simulink model "VMO_GP"  (R2021a)
settings: Solver=VariableStepAuto  StartTime=0.0  StopTime=50  FixedStep=0.001  RelTol=1e-3
model workspace (MAT data in the model file):
  lambda = 20
  po = [0  0  0.5; 0.5  0  0; 0  0  -0.5; -0.5  0  0]
undefined symbols (not defined in the file or in its folder): mergepose
libraries: simlib_vpc_basic x4, simlib_vpc_coremath x2, simlib_vpc_gp x1
settings Model: Creator=marco  LastModifiedBy=marco
settings SolverCC: AlgebraicLoopSolver=TrustRegion
settings DebuggingCC: AlgebraicLoopMsg=none  SFMachineParentedDataDiag=warning
settings RTWCC: Toolchain=Clang v3.1 | gmake (64-bit Mac)

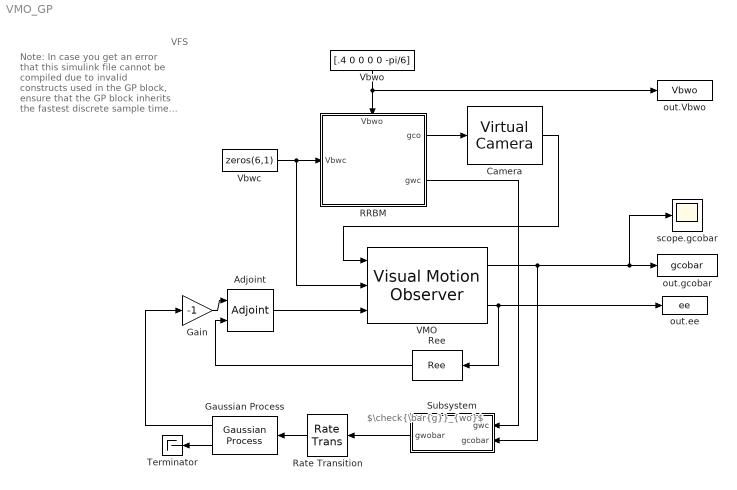
== system VMO_GP ==
  note: VFS
  note: $\check{\bar{g}}_{wo}$
  note: Note:
      |
      | In case you get an error that this simulink file cannot be compiled due to invalid constructs used in the GP block, ensure that the GP block inherits the fastest discrete sample time if you use a variable step solver!
      |
      | Simulink sometimes tends to forget this setting if the file has been altered by library block updates...
  Adjoint : simlib_vpc_basic/Adjoint  adjointtype=orientation
      settings: SourceProductName=VPC Library
  Camera : simlib_vpc_basic/Virtual Camera  camtype=Pinhole  po=po  lambda=lambda
      settings: SourceProductName=VPC Library
  Gain : Gain  Gain=-1
  Gaussian Process : simlib_vpc_gp/Gaussian Process  X=[0.630556779825130,-1.35266887136097,0.100000000000000,0,0,-2.69410960293706;-0.463678144695271,-0.643799212064173,0.100000000000000,0,0,1.54442416387410;0.824727377358984,-1.21916548494542,0.100000000000000,0,0,-2.38442385676060;-0.452218900404542,-0.797273527670285,0.100000000000000,0,0,1.74622300936847;0.0735614873622379,-1.39355710178978,0.100000000000000,0,0,2.84066394855618;1.02709161361236,-0.429534249029276,0.100000000000000,0,0,-1.25892388595008;0.466856822301989,0.0815553296307524,0.100000000000000,0,0,-0.220190026018465;0.700684091841969,-0.0135113083777034,0.100000000000000,0,0,-0.552120963315916;-0.371594765405859,-0.299841291908943,0.100000000000000,0,0,1.07400302698064;0.493112507590971,0.0751893431225574,0.100000000000000,0,0,-0.255556274277872;0.281774950670647,-1.42767003232909,0.100000000000000,0,0,3.11773385638550;0.454855984665292,0.0841403324164895,0.100000000000000,0,0,-0.204120492121210;-0.415643299934273,-0.931272694722223,0.100000000000000,0,0,1.92829566524218;-0.463704413816322,-0.644822651287869,0.100000000000000,0,0,1.54576428394557;0.556071793384051,0.0558043832070477,0.100000000000000,0,0,-0.341814497897213;0.693810642313243,-1.31856056106307,0.100000000000000,0,0,-2.60000519109390;0.139429262029952,-1.41082195312738,0.100000000000000,0,0,2.92982683484421;0.225444734023850,-1.42424078855668,0.100000000000000,0,0,3.04384446142033;0.336503259664140,0.0991274476359257,0.100000000000000,0,0,-0.0478008530352022;-0.0531708161840424,-1.34135090449317,0.100000000000000,0,0,2.66100597056373]  Y=[0.400400483777776,6.20811263679909e-05,-0.000162652488464400,-0.000273446486135386,-0.000116687704346113,-0.523637613189225;0.399798663298112,6.11577178236449e-05,-1.83837233443192e-05,-5.72316425158164e-06,6.14391667114607e-05,-0.523595018762085;0.399925527207886,0.000102384004761238,-1.86739670271565e-05,-7.65017896653280e-06,1.02416118127720e-05,-0.523520368962881;0.399947525768678,-1.43211998020437e-05,3.27587119859464e-05,0.000113295220747682,-3.51700486357816e-05,-0.523531017064327;0.400111825354472,3.90999913623867e-05,5.26454668989892e-05,-9.40761215372331e-06,-4.25671711451752e-05,-0.523522634661440;0.399825833671039,-7.77258024196419e-05,-0.000206163047832629,6.59457899046355e-06,-8.22951844090592e-05,-0.523698419763352;0.399974962089588,-1.88854060648864e-05,3.09965613525548e-05,0.000245980243067202,-0.000217647213137394,-0.523689484439025;0.400074095697642,-1.41829641564855e-05,4.84335658930588e-05,4.75025873122616e-05,-9.10729403185158e-05,-0.523588569617585;0.400083248675279,0.000132443300246046,-0.000157442907631115,-2.83480572397296e-05,-4.51136693628445e-07,-0.523633397263088;0.400032876833907,6.44379360130703e-05,-0.000128770670171243,1.64273840062151e-05,-5.42887023463567e-05,-0.523597545840270;0.399861552080262,4.56874083328404e-06,7.00785975750203e-05,-6.15101314259443e-07,4.31078905663889e-05,-0.523618963169823;0.399914551858832,-2.55383556669599e-05,-1.30390132312550e-06,7.61551335297795e-05,6.91286456425908e-05,-0.523720317431230;0.399989694796018,-9.69835284456510e-05,-0.000159624446683547,5.99762161919923e-05,0.000131711278614893,-0.523655772898916;0.400222298778977,-0.000246033432409541,0.000124299539566767,-0.000133706441116990,-2.05671749582727e-05,-0.523700638665687;0.399762190818026,-6.58016860859998e-05,-0.000101273579864964,-4.49734662190949e-05,-4.24077389374409e-05,-0.523699857561119;0.399890067610248,8.46601373619946e-05,0.000103500553198445,2.49750235544482e-05,-0.000122935827076731,-0.523757337794273;0.400083233949163,-8.14595746369251e-05,6.44687411206958e-05,-3.23632580436771e-05,5.02141191648383e-05,-0.523497516354906;0.400296665626679,4.06352239193496e-05,1.07765346007298e-05,9.65656080285521e-05,-6.27072577361815e-05,-0.523553573528897;0.400010008726827,-1.62468044620332e-06,-9.59528973827606e-06,-0.000138103359704066,1.33199410225313e-05,-0.523641337975467;0.400029450602431,-0.000122327126645188,0.000161646482165890,-0.000230740252290899,7.19352758249854e-05,-0.523425710873170]  sigman=1e-2.*ones(6,1)  kernel=Squared Exponential ARD  hyp=[168349.386723878,4375.40145868387,1,1,1,479344.764312913,0.399829624229871;28.6402467014848,24.0814787639094,1,1,1,805.684470437413,2.45252270103894e-11;108.279817332599,159.557667315089,1,1,1,114449.667169593,3.58973817196935e-12;36.4794037030670,12.8797220031653,1,1,1,5438.09149501526,4.41867700247680e-09;2.19447546863541,62.6618892840448,1,1,1,8349.10365718305,1.24554979865875e-05;6611001.04652391,10465.6546012474,1,1,1,35776.6715743359,0.523405437753361]
      settings: SourceProductName=VPC Library
  RRBM : Subsystem
      settings: PortSchema="{\"entries\":[{\"content\":{\"sides\":[{\"content\":{\"connectorIds\":[\"In1\"]},\"type\":\"ConnectorPlacement.EquallySpacedRectSide\",\"uuid\":\"ce1006a6-ff18-4db7-ad69-3a60144a672f\"},{\"content\":{\"connectorIds\":[\"Out1\",\"Out2\"],\"side\":\"RIGHT\"},\"type\":\"ConnectorPlacement.EquallySpacedRectSide\",\"uuid\":\"9f6b7cf2-eb23-4db0-862a-f9244538bf77\"},{\"content\":{\"connectorIds\":[\"In2\"],\"side\":\"TOP\"},\"type\":\"ConnectorPlacement.EquallySpacedRectSide\",\"uuid\":\"e4abfdaf-0145-4439-9abb-46234dad4713\"},{\"content\":{\"connectorIds\":[],\"side\":\"HIDDEN\"},\"type\":\"ConnectorPlacement.EquallySpacedRectSide\",\"uuid\":\"77f0040d-d5e2-4b47-95e1-996605172696\"}]},\"type\":\"ConnectorPlacement.EquallySpacedConnector\",\"uuid\":\"a30e6cf8-5cfd-45cc-9c7f-0b16cc268ba1\"}],\"packageUris\":[\"http://schema.mathworks.com/mf0/Connector/R2020b\"],\"version\":\"1.0\"}"
      mask Display:
      | % Glitch in Matlab: If you define a line whose starting point and end point
      | % is equal, then the entire mask block is plotted in bold
      | plot([0,0],[0,0])
      | 
      | % Draw Box
      | plot([0,1,1,0,0],[0,0,1,1,0])
      | 
      | % Write label
      | fprintf('1 Agent\n1 Target','texmode','on')
      | 
      | % Label ports
      | port_label('input',1,'V^{b}_{wc}','texmode','on')
      | port_label('input',2,'V^{b}_{wo}','texmode','on')
      | port_label('output',1,'g_{co}','texmode','on')
      | port_label('output',2,'g_{wc}','texmode','on')
  Rate Transition : RateTransition
  Ree : simlib_vpc_coremath/Ree
      settings: SourceProductName=VPC Library
  Subsystem : Subsystem
      mask Display:
      | % Write label
      | % disp('Trans','texmode','on')
      | 
      | % Label ports
      | port_label('input',1,'g_{wc}','texmode','on')
      | port_label('input',2,'g_{co,bar}','texmode','on')
      | port_label('output',1,'g^{\upsilon}_{wo,bar}','texmode','on')
  Terminator : Terminator
  VMO : simlib_vpc_basic/Visual Motion Observer  gcobar0=mergepose(eye(3),[0 1 0])  projection=on  Ke_source=internal  Ke=5*eye(6)  show_ue_aux=on  show_ee=on  show_dgcobar=off  camtype=Pinhole  fo=po  lambda=lambda
      settings: SourceProductName=VPC Library
  Vbwc : Constant  Value=zeros(6,1)
  Vbwo : Constant  Value=[.4 0 0 0 0 -pi/6]
  out.Vbwo : ToWorkspace  VariableName=Vbwo  SaveFormat=Structure With Time  SampleTime=-1
  out.ee : ToWorkspace  VariableName=ee  SaveFormat=Structure With Time  SampleTime=-1
  out.gcobar : ToWorkspace  VariableName=gcobar  SaveFormat=Structure With Time  SampleTime=-1
  scope.gcobar : Scope
  wires:
  Vbwc/1 -> RRBM/1(Vbwc), VMO/2
  Vbwo/1 -> RRBM/2(Vbwo), out.Vbwo/1
  RRBM/1(gco) -> Camera/1
  VMO/2 -> out.ee/1, Ree/1
  Camera/1 -> VMO/1
  VMO/1 -> Subsystem/2(gcobar), scope.gcobar/1, out.gcobar/1
  Gaussian Process/2 -> Terminator/1
  Gain/1 -> Adjoint/1
  Adjoint/1 -> VMO/3
  Ree/1 -> Adjoint/2
  Gaussian Process/1 -> Gain/1
  RRBM/2(gwc) -> Subsystem/1(gwc)
  Subsystem/1(gwobar) -> Rate Transition/1
  Rate Transition/1 -> Gaussian Process/1

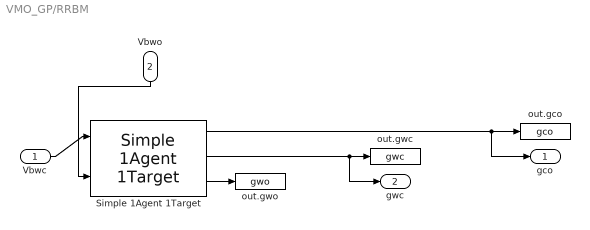
== system VMO_GP/RRBM ==
  Vbwc : Inport
  Vbwo : Inport  Port=2
  Simple 1Agent 1Target : simlib_vpc_basic/Simple 1Agent 1Target  gwc0=mergepose(eye(3),[0 -5 0])  projectionAgent=on  gwo0=mergepose(eye(3),[0.3 0.1 0.1])  projectionTarget=on  showgwc=on  showdgwc=off  showgwo=on  showdgwo=off
      settings: SourceProductName=VPC Library
  out.gco : ToWorkspace  VariableName=gco  SaveFormat=Structure With Time  SampleTime=-1
  out.gwc : ToWorkspace  VariableName=gwc  SaveFormat=Structure With Time  SampleTime=-1
  out.gwo : ToWorkspace  VariableName=gwo  SaveFormat=Structure With Time  SampleTime=-1
  gco : Outport
  gwc : Outport  Port=2
  wires:
  Vbwo/1 -> Simple 1Agent 1Target/2
  Vbwc/1 -> Simple 1Agent 1Target/1
  Simple 1Agent 1Target/2 -> gwc/1, out.gwc/1
  Simple 1Agent 1Target/3 -> out.gwo/1
  Simple 1Agent 1Target/1 -> gco/1, out.gco/1

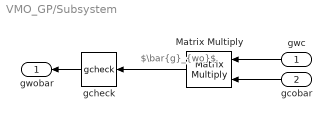
== system VMO_GP/Subsystem ==
  note: $\bar{g}_{wo}$
  gwc : Inport
  gcobar : Inport  Port=2
  Matrix Multiply : Product  Multiplication=Matrix(*)
  gcheck : simlib_vpc_coremath/gcheck
      settings: SourceProductName=VPC Library
  gwobar : Outport
  wires:
  gwc/1 -> Matrix Multiply/1
  gcobar/1 -> Matrix Multiply/2
  Matrix Multiply/1 -> gcheck/1
  gcheck/1 -> gwobar/1
